simulink model "SV16"  (R2026a)
settings: Solver=VariableStepAuto  StopTime=0.1
libraries: simulink x55, hdlsllib x34
(part 2 of 2)

== system SV16/INSTRUCTION_MEMORY/MEMORY_BANK_8_B0/R4 ==
  D : Inport
  WE : Inport  Port=2
  Reset : Inport  Port=3
  Constant : Constant  Value=0  OutDataTypeStr=uint16
  Constant1 : Constant  OutDataTypeStr=uint16
  Switch : Switch  Criteria=u2 > Threshold  SaturateOnIntegerOverflow=off  InputSameDT=off
  Switch1 : Switch  Criteria=u2 > Threshold  SaturateOnIntegerOverflow=off  InputSameDT=off
  Unit Delay Enabled Synchronous : hdlsllib/Discrete/Unit Delay Enabled Synchronous  InitialCondition=0.0  SampleTime=-1
  D4 : Outport
  wires:
  D/1 -> Switch/1
  WE/1 -> Switch/2
  Unit Delay Enabled Synchronous/1 -> D4/1, Switch/3
  Reset/1 -> Switch1/2
  Constant/1 -> Switch1/1
  Switch/1 -> Switch1/3
  Switch1/1 -> Unit Delay Enabled Synchronous/1
  Constant1/1 -> Unit Delay Enabled Synchronous/2

== system SV16/INSTRUCTION_MEMORY/MEMORY_BANK_8_B0/R5 ==
  D : Inport
  WE : Inport  Port=2
  Reset : Inport  Port=3
  Constant : Constant  Value=0  OutDataTypeStr=uint16
  Constant1 : Constant  OutDataTypeStr=uint16
  Switch : Switch  Criteria=u2 > Threshold  SaturateOnIntegerOverflow=off  InputSameDT=off
  Switch1 : Switch  Criteria=u2 > Threshold  SaturateOnIntegerOverflow=off  InputSameDT=off
  Unit Delay Enabled Synchronous : hdlsllib/Discrete/Unit Delay Enabled Synchronous  InitialCondition=0.0  SampleTime=-1
  D5 : Outport
  wires:
  D/1 -> Switch/1
  WE/1 -> Switch/2
  Unit Delay Enabled Synchronous/1 -> D5/1, Switch/3
  Reset/1 -> Switch1/2
  Constant/1 -> Switch1/1
  Switch/1 -> Switch1/3
  Switch1/1 -> Unit Delay Enabled Synchronous/1
  Constant1/1 -> Unit Delay Enabled Synchronous/2

== system SV16/INSTRUCTION_MEMORY/MEMORY_BANK_8_B0/R6 ==
  D : Inport
  WE : Inport  Port=2
  Reset : Inport  Port=3
  Constant : Constant  Value=0  OutDataTypeStr=uint16
  Constant1 : Constant  OutDataTypeStr=uint16
  Switch : Switch  Criteria=u2 > Threshold  SaturateOnIntegerOverflow=off  InputSameDT=off
  Switch1 : Switch  Criteria=u2 > Threshold  SaturateOnIntegerOverflow=off  InputSameDT=off
  Unit Delay Enabled Synchronous : hdlsllib/Discrete/Unit Delay Enabled Synchronous  InitialCondition=0.0  SampleTime=-1
  D6 : Outport
  wires:
  D/1 -> Switch/1
  WE/1 -> Switch/2
  Unit Delay Enabled Synchronous/1 -> D6/1, Switch/3
  Reset/1 -> Switch1/2
  Constant/1 -> Switch1/1
  Switch/1 -> Switch1/3
  Switch1/1 -> Unit Delay Enabled Synchronous/1
  Constant1/1 -> Unit Delay Enabled Synchronous/2

== system SV16/INSTRUCTION_MEMORY/MEMORY_BANK_8_B0/R7 ==
  D : Inport
  WE : Inport  Port=2
  Reset : Inport  Port=3
  Constant : Constant  Value=0  OutDataTypeStr=uint16
  Constant1 : Constant  OutDataTypeStr=uint16
  Switch : Switch  Criteria=u2 > Threshold  SaturateOnIntegerOverflow=off  InputSameDT=off
  Switch1 : Switch  Criteria=u2 > Threshold  SaturateOnIntegerOverflow=off  InputSameDT=off
  Unit Delay Enabled Synchronous : hdlsllib/Discrete/Unit Delay Enabled Synchronous  InitialCondition=0.0  SampleTime=-1
  D7 : Outport
  wires:
  D/1 -> Switch/1
  WE/1 -> Switch/2
  Unit Delay Enabled Synchronous/1 -> D7/1, Switch/3
  Reset/1 -> Switch1/2
  Constant/1 -> Switch1/1
  Switch/1 -> Switch1/3
  Switch1/1 -> Unit Delay Enabled Synchronous/1
  Constant1/1 -> Unit Delay Enabled Synchronous/2

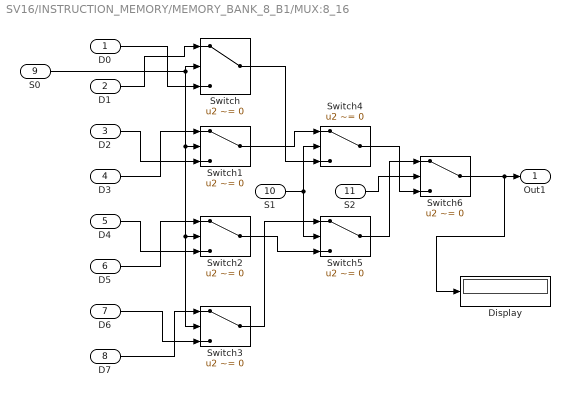
== system SV16/INSTRUCTION_MEMORY/MEMORY_BANK_8_B1/MUX:8_16 ==
  D0 : Inport  OutDataTypeStr=uint32
  D1 : Inport  Port=2  OutDataTypeStr=uint32
  D2 : Inport  Port=3  OutDataTypeStr=uint32
  D3 : Inport  Port=4  OutDataTypeStr=uint32
  D4 : Inport  Port=5  OutDataTypeStr=uint32
  D5 : Inport  Port=6  OutDataTypeStr=uint32
  D6 : Inport  Port=7  OutDataTypeStr=uint32
  D7 : Inport  Port=8  OutDataTypeStr=uint32
  S0 : Inport  Port=9  OutDataTypeStr=boolean
  S1 : Inport  Port=10  OutDataTypeStr=boolean
  S2 : Inport  Port=11  OutDataTypeStr=boolean
  Display : Display
  Switch{,1..6} (7 alike) : Switch  Criteria=u2 ~= 0  SaturateOnIntegerOverflow=off  InputSameDT=off
  Out1 : Outport  OutDataTypeStr=uint32
  wires:
  D0/1 -> Switch/3
  S0/1 -> Switch/2, Switch3/2, Switch2/2, Switch1/2
  D3/1 -> Switch1/1
  D5/1 -> Switch2/1
  D6/1 -> Switch3/3
  Switch/1 -> Switch4/3
  S1/1 -> Switch5/2, Switch4/2
  S2/1 -> Switch6/2
  Switch6/1 -> Display/1, Out1/1
  D1/1 -> Switch/1
  D2/1 -> Switch1/3
  D4/1 -> Switch2/3
  D7/1 -> Switch3/1
  Switch4/1 -> Switch6/3
  Switch5/1 -> Switch6/1
  Switch1/1 -> Switch4/1
  Switch2/1 -> Switch5/3
  Switch3/1 -> Switch5/1

== system SV16/INSTRUCTION_MEMORY/MEMORY_BANK_8_B1/R0 ==
  D : Inport
  WE : Inport  Port=2
  Reset : Inport  Port=3
  Constant : Constant  Value=0  OutDataTypeStr=uint16
  Constant1 : Constant  OutDataTypeStr=uint32
  Subsystem : Subsystem
  Switch : Switch  Criteria=u2 > Threshold  SaturateOnIntegerOverflow=off  InputSameDT=off
  Switch1 : Switch  Criteria=u2 > Threshold  SaturateOnIntegerOverflow=off  InputSameDT=off
  D0 : Outport  OutDataTypeStr=uint32
  wires:
  D/1 -> Switch/1
  WE/1 -> Switch/2
  Reset/1 -> Switch1/2
  Constant/1 -> Switch1/1
  Switch/1 -> Switch1/3
  Subsystem/1(y) -> D0/1, Switch/3
  Switch1/1 -> Subsystem/1(u)
  Constant1/1 -> Subsystem/2(E)

== system SV16/INSTRUCTION_MEMORY/MEMORY_BANK_8_B1/R1 ==
  D : Inport
  WE : Inport  Port=2
  Reset : Inport  Port=3
  Constant : Constant  Value=0  OutDataTypeStr=uint16
  Constant1 : Constant  OutDataTypeStr=uint16
  Switch : Switch  Criteria=u2 > Threshold  SaturateOnIntegerOverflow=off  InputSameDT=off
  Switch1 : Switch  Criteria=u2 > Threshold  SaturateOnIntegerOverflow=off  InputSameDT=off
  Unit Delay Enabled Synchronous : hdlsllib/Discrete/Unit Delay Enabled Synchronous  InitialCondition=0.0  SampleTime=-1
  D1 : Outport
  wires:
  D/1 -> Switch/1
  WE/1 -> Switch/2
  Unit Delay Enabled Synchronous/1 -> D1/1, Switch/3
  Reset/1 -> Switch1/2
  Constant/1 -> Switch1/1
  Switch/1 -> Switch1/3
  Switch1/1 -> Unit Delay Enabled Synchronous/1
  Constant1/1 -> Unit Delay Enabled Synchronous/2

== system SV16/INSTRUCTION_MEMORY/MEMORY_BANK_8_B1/R2 ==
  D : Inport
  WE : Inport  Port=2
  Reset : Inport  Port=3
  Constant : Constant  Value=0  OutDataTypeStr=uint16
  Constant1 : Constant  OutDataTypeStr=uint16
  Switch : Switch  Criteria=u2 > Threshold  SaturateOnIntegerOverflow=off  InputSameDT=off
  Switch1 : Switch  Criteria=u2 > Threshold  SaturateOnIntegerOverflow=off  InputSameDT=off
  Unit Delay Enabled Synchronous : hdlsllib/Discrete/Unit Delay Enabled Synchronous  InitialCondition=0.0  SampleTime=-1
  D2 : Outport
  wires:
  D/1 -> Switch/1
  WE/1 -> Switch/2
  Unit Delay Enabled Synchronous/1 -> D2/1, Switch/3
  Reset/1 -> Switch1/2
  Constant/1 -> Switch1/1
  Switch/1 -> Switch1/3
  Switch1/1 -> Unit Delay Enabled Synchronous/1
  Constant1/1 -> Unit Delay Enabled Synchronous/2

== system SV16/INSTRUCTION_MEMORY/MEMORY_BANK_8_B1/R3 ==
  D : Inport
  WE : Inport  Port=2
  Reset : Inport  Port=3
  Constant : Constant  Value=0  OutDataTypeStr=uint16
  Constant1 : Constant  OutDataTypeStr=uint16
  Switch : Switch  Criteria=u2 > Threshold  SaturateOnIntegerOverflow=off  InputSameDT=off
  Switch1 : Switch  Criteria=u2 > Threshold  SaturateOnIntegerOverflow=off  InputSameDT=off
  Unit Delay Enabled Synchronous : hdlsllib/Discrete/Unit Delay Enabled Synchronous  InitialCondition=0.0  SampleTime=-1
  D3 : Outport
  wires:
  D/1 -> Switch/1
  WE/1 -> Switch/2
  Unit Delay Enabled Synchronous/1 -> D3/1, Switch/3
  Reset/1 -> Switch1/2
  Constant/1 -> Switch1/1
  Switch/1 -> Switch1/3
  Switch1/1 -> Unit Delay Enabled Synchronous/1
  Constant1/1 -> Unit Delay Enabled Synchronous/2

== system SV16/INSTRUCTION_MEMORY/MEMORY_BANK_8_B1/R4 ==
  D : Inport
  WE : Inport  Port=2
  Reset : Inport  Port=3
  Constant : Constant  Value=0  OutDataTypeStr=uint16
  Constant1 : Constant  OutDataTypeStr=uint16
  Switch : Switch  Criteria=u2 > Threshold  SaturateOnIntegerOverflow=off  InputSameDT=off
  Switch1 : Switch  Criteria=u2 > Threshold  SaturateOnIntegerOverflow=off  InputSameDT=off
  Unit Delay Enabled Synchronous : hdlsllib/Discrete/Unit Delay Enabled Synchronous  InitialCondition=0.0  SampleTime=-1
  D4 : Outport
  wires:
  D/1 -> Switch/1
  WE/1 -> Switch/2
  Unit Delay Enabled Synchronous/1 -> D4/1, Switch/3
  Reset/1 -> Switch1/2
  Constant/1 -> Switch1/1
  Switch/1 -> Switch1/3
  Switch1/1 -> Unit Delay Enabled Synchronous/1
  Constant1/1 -> Unit Delay Enabled Synchronous/2

== system SV16/INSTRUCTION_MEMORY/MEMORY_BANK_8_B1/R5 ==
  D : Inport
  WE : Inport  Port=2
  Reset : Inport  Port=3
  Constant : Constant  Value=0  OutDataTypeStr=uint16
  Constant1 : Constant  OutDataTypeStr=uint16
  Switch : Switch  Criteria=u2 > Threshold  SaturateOnIntegerOverflow=off  InputSameDT=off
  Switch1 : Switch  Criteria=u2 > Threshold  SaturateOnIntegerOverflow=off  InputSameDT=off
  Unit Delay Enabled Synchronous : hdlsllib/Discrete/Unit Delay Enabled Synchronous  InitialCondition=0.0  SampleTime=-1
  D5 : Outport
  wires:
  D/1 -> Switch/1
  WE/1 -> Switch/2
  Unit Delay Enabled Synchronous/1 -> D5/1, Switch/3
  Reset/1 -> Switch1/2
  Constant/1 -> Switch1/1
  Switch/1 -> Switch1/3
  Switch1/1 -> Unit Delay Enabled Synchronous/1
  Constant1/1 -> Unit Delay Enabled Synchronous/2

== system SV16/INSTRUCTION_MEMORY/MEMORY_BANK_8_B1/R6 ==
  D : Inport
  WE : Inport  Port=2
  Reset : Inport  Port=3
  Constant : Constant  Value=0  OutDataTypeStr=uint16
  Constant1 : Constant  OutDataTypeStr=uint16
  Switch : Switch  Criteria=u2 > Threshold  SaturateOnIntegerOverflow=off  InputSameDT=off
  Switch1 : Switch  Criteria=u2 > Threshold  SaturateOnIntegerOverflow=off  InputSameDT=off
  Unit Delay Enabled Synchronous : hdlsllib/Discrete/Unit Delay Enabled Synchronous  InitialCondition=0.0  SampleTime=-1
  D6 : Outport
  wires:
  D/1 -> Switch/1
  WE/1 -> Switch/2
  Unit Delay Enabled Synchronous/1 -> D6/1, Switch/3
  Reset/1 -> Switch1/2
  Constant/1 -> Switch1/1
  Switch/1 -> Switch1/3
  Switch1/1 -> Unit Delay Enabled Synchronous/1
  Constant1/1 -> Unit Delay Enabled Synchronous/2

== system SV16/INSTRUCTION_MEMORY/MEMORY_BANK_8_B1/R7 ==
  D : Inport
  WE : Inport  Port=2
  Reset : Inport  Port=3
  Constant : Constant  Value=0  OutDataTypeStr=uint16
  Constant1 : Constant  OutDataTypeStr=uint16
  Switch : Switch  Criteria=u2 > Threshold  SaturateOnIntegerOverflow=off  InputSameDT=off
  Switch1 : Switch  Criteria=u2 > Threshold  SaturateOnIntegerOverflow=off  InputSameDT=off
  Unit Delay Enabled Synchronous : hdlsllib/Discrete/Unit Delay Enabled Synchronous  InitialCondition=0.0  SampleTime=-1
  D7 : Outport
  wires:
  D/1 -> Switch/1
  WE/1 -> Switch/2
  Unit Delay Enabled Synchronous/1 -> D7/1, Switch/3
  Reset/1 -> Switch1/2
  Constant/1 -> Switch1/1
  Switch/1 -> Switch1/3
  Switch1/1 -> Unit Delay Enabled Synchronous/1
  Constant1/1 -> Unit Delay Enabled Synchronous/2

== system SV16/INSTRUCTION_MEMORY/MEMORY_BANK_8_B0/R0/Subsystem ==
  u : Inport
  E : Inport  Port=2  OutDataTypeStr=uint32
  Unit Delay Enabled Synchronous : hdlsllib/Discrete/Unit Delay Enabled Synchronous  InitialCondition=0.0  SampleTime=-1
  y : Outport
  wires:
  Unit Delay Enabled Synchronous/1 -> y/1
  E/1 -> Unit Delay Enabled Synchronous/2
  u/1 -> Unit Delay Enabled Synchronous/1

== system SV16/INSTRUCTION_MEMORY/MEMORY_BANK_8_B1/R0/Subsystem ==
  u : Inport
  E : Inport  Port=2  OutDataTypeStr=uint32
  Unit Delay Enabled Synchronous : hdlsllib/Discrete/Unit Delay Enabled Synchronous  InitialCondition=0.0  SampleTime=-1
  y : Outport
  wires:
  Unit Delay Enabled Synchronous/1 -> y/1
  E/1 -> Unit Delay Enabled Synchronous/2
  u/1 -> Unit Delay Enabled Synchronous/1
